simulink model "Winkelsensor"  (R2021a)
settings: Solver=ode3  StartTime=0.0  StopTime=10  FixedStep=0.01  RelTol=1e-3
settings Model: Creator=Oceaner  LastModifiedBy=Oceaner

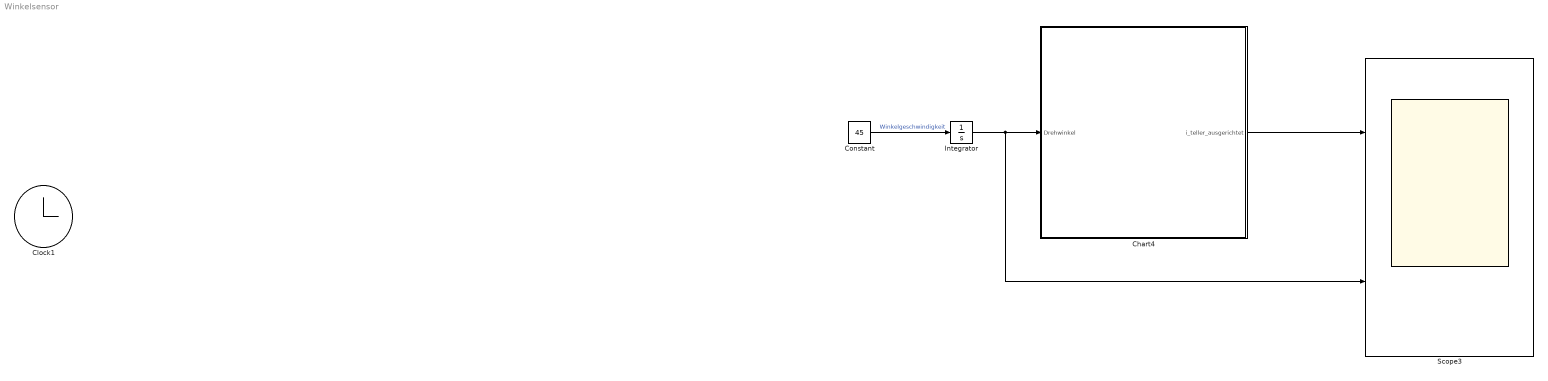
== system Winkelsensor ==
  Chart4 : Stateflow chart  TreatAsAtomicUnit=on
  Clock1 : Clock
  Constant : Constant  Value=45
  Integrator : Integrator
  Scope3 : Scope  NumInputPorts=2
  wires:
  Chart4/1(i_teller_ausgerichtet) -> Scope3/1
  Constant/1 -> Integrator/1  "Winkelgeschwindigkeit"
  Integrator/1 -> Scope3/2, Chart4/1(Drehwinkel)

== stateflow chart Winkelsensor/Chart4 ==
  state pause
    en:i_teller_ausgerichtet=1;
  state N
    en:i_teller_ausgerichtet=0;
  pause -> N : [mod(Drehwinkel,90)>2&&mod(Drehwinkel,90)<88]
  N -> pause : [(mod(Drehwinkel,90)>=0&&mod(Drehwinkel,90)<=2)||(mod(Drehwinkel,90)>=88&&mod(Drehwinkel,90)<=90)]
  (default) -> N
  data: Drehwinkel input; i_teller_ausgerichtet output
